simulink model "control_ejemplo"  (R2018a)
settings: Solver=VariableStepAuto  StartTime=0.0  StopTime=100  RelTol=1e-3
libraries: cstblocks x2
settings Model: Creator=xndyl  LastModifiedBy=xndyl

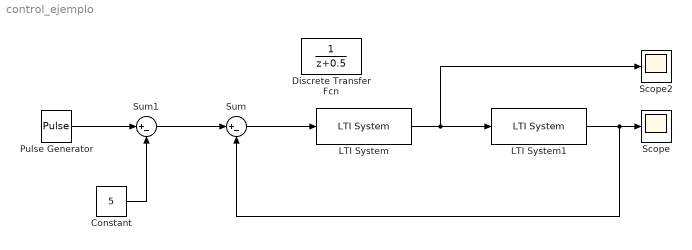
== system control_ejemplo ==
  Constant : Constant  Value=5
  Discrete Transfer Fcn : DiscreteTransferFcn
  LTI System : cstblocks/LTI System  sys=Cd  IC=[]
  LTI System1 : cstblocks/LTI System  sys=G_total  IC=[]
  Pulse Generator : DiscretePulseGenerator  PulseType=Time based  Amplitude=10  Period=20  PulseWidth=50
  Scope : Scope
  Scope2 : Scope
  Sum : Sum  Inputs=|+-
  Sum1 : Sum  Inputs=|+-
  wires:
  LTI System/1 -> Scope2/1, LTI System1/1
  LTI System1/1 -> Sum/2, Scope/1
  Sum/1 -> LTI System/1
  Sum1/1 -> Sum/1
  Pulse Generator/1 -> Sum1/1
  Constant/1 -> Sum1/2
